simulink model "MicrogridControl"  (R2025b)
settings: Solver=VariableStepAuto  StartTime=0.0  StopTime=8  FixedStep=Ts  RelTol=1e-3
PreLoadFcn:
  | NormalOperation;
  | MicrogridControlParam;
undefined symbols (not defined in the file): base, bessModeInitial, bessSystem, bessVoltage, breakerStatus, DiscIntNeverNeededParam, ee_sli_rtmsupport, event, gcbh, generator, gflInverter, gfmInverter, Inertia, lineInductance, lineResistance, machine, plannedIsland, pmsm, powerLimit, powerQuality, PV, PVInverter, ref, resync, solar, solarInsolationChange, systemFrequency, Ts, windController, windSystem, windTurbine
libraries: nesl_utility x234, ee_lib x174, fl_lib x143, eeGeneralControl x137, simulink x78, eeTransforms x47, slpidlib x23, nesl_utility_internal x12, eePwmGenerator x9, eeSinusoidalMeasurementV2 x9, custom_lib x7, batteryecm_lib x6
(part 12 of 25)

== system MicrogridControl/Wind Farm/Wind Plant Integrated/Detailed/Wind Turbine and Converters ==
  note: Plant
  note: Controller
  pitch : Inport
  Wind_speed : Inport  Port=2
  LVRT : Inport  Port=3
  QRef : Inport  Port=4
  VIBus : Inport  Port=5
  Signal Conditioning : Subsystem
  Wind Controller : Subsystem  mask(Wind Controller){baseVac=Vac, baseImpedance=Vac^2/(plantRating*1000)%base.impedance, basePower=plantRating*1000, inductance=filterInductance, capacitance=0.1, Vdc=baseVoltageDC, frequency=frequency, iMaxPU=iMaxPU, mpptPower=windSystem.mpptPower, mpptWindSpeed=windSystem.mpptWindSpeed, p=p, psim=psim, Rs=Rs, Ld=Ld, Lq=Lq, airDensity=airDensity, turbineRadius=turbineRadius, pitch=pitch, TSR=TSR, cp=cp, wt=wt, rt=wt, Inertia=200, Kp_dc=windController.kpVoltage, Ki_dc=windController.kiVoltage, Kdpi_g=windController.kpId, Kdii_g=windController.kiId, Kqpi_g=windController.kpIq, Kqii_g=windController.kiIq, Kdip_sm=windController.kpMSC, Kdii_sm=windController.kiMSC, Kqip_sm=windController.kpMSC, Kqii_sm=windController.kiMSC}
      mask prompts: baseVac "Base AC Voltage (V)"; baseImpedance "Base Impedance (Ohm)"; basePower "Base Power (W)"; inductance "Filter Inductance (H)"; capacitance "DC bus capacitance (F)"; Vdc "DC bus Voltage (V)"; frequency "System Frequency (Hz)"; iMaxPU "Maximum Current (pu)"; mpptPower "MPPT Power"; mpptWindSpeed "MPPT Wind Speed"; p "Number of pole pairs"; psim "PMSM flux linkage"; Rs "Stator resistance (Ohm)"; Ld "Stator d-axis inductance (H)"; Lq "Stator q-axis inductance (H)"; airDensity "Air Density (kg/m^3)"; turbineRadius "Turbine radius (m)"; pitch "Pitch angle vector (deg)"; cp "Power Coefficient (cp)"; wt "Wind velocity threshold (m/s)"; rt "Rotational velocity threshold (rad/s)"; Inertia "Turbine Inertia (kgm^2)"; Kp_dc "Proportional gain"; Ki_dc "Integral gain"; Kdpi_g "d-axis proportional gain"; Kdii_g "d-axis integrall gain"; Kqpi_g "q-axis proportional gain"; Kqii_g "q-axis integral gain"; Kdip_sm "d-axis proportional gain"; Kdii_sm "d-axis integral gain"; Kqip_sm "q-axis proportional gain"; Kqii_sm "q-axis integral gain"
      mask help: This block implements the control strategy for a Type-4 wind turbine system, which uses a full-scale back-to-back converter to interface the generator with the grid. The controller manages both the machine-side converter (for generator torque and speed control) and the grid-side converter (for active/reactive power regulation and grid compliance). It ensures smooth power transfer, grid code adherence, and dynamic performance under varying wind and grid conditions. The design supports advanced functionalities such as fault ride-through and voltage support.
      mask DialogControl Container9 Prompt: General
      mask DialogControl Container3 Prompt: PMSM Parameters
      mask DialogControl Container4 Prompt: Wind Turbine Parameters
      mask DialogControl Container6 Prompt: Grid Side Converter Controller
      mask DialogControl Container7 Prompt: DC bus voltage controller
      mask DialogControl Container8 Prompt: Current Controller
      mask DialogControl Container10 Prompt: Machine Side Converter Controller
  Wind Plant : Subsystem  mask(Wind Plant){ratedVoltage=Vac, Vdc=baseVoltageDC, capDC=capacitance, airDensity=airDensity, turbineRadius=turbineRadius, pitch=pitch, TSR=TSR, cp=cp, wt=wt, rt=rt, p=p, psim=psim, Rs=Rs, Ld=Ld, Lq=Lq, converterFidelity=Average, fSw=fSw}
      mask prompts: ratedVoltage "Rated voltage on AC side (V)"; Vdc "DC bus violtage (V)"; capDC "DC bus capacitance (F)"; airDensity "Air density (kg/m^3)"; turbineRadius "Turbine radius (m)"; pitch "Pitch angle vector (deg)"; TSR "Tip speed ratio"; cp "Power coefficient table, Cp(beta,TSR)"; wt "Wind velocity threshold (m/s)"; rt "Rotational velocity threshold (rad/s)"; p "Number of pole pairs"; psim "PMSM flux linkage (Wb)"; Rs "Stator resistance (Ohm)"; Ld "Stator d-axis inductance (H)"; Lq "Stator q-axis inductance (H)"; converterFidelity "Converter Fidelity"; fSw "Switching Frequency (kHz)"
      mask help: This block represents the physical interface between the wind turbine and the power converters. It models the electrical and dynamic characteristics of the wind turbine connected to a converter, while expecting an external control signal for operation
      settings: CopyFcn=set_param(gcbh,'LinkStatus','none');
      mask TypeOptions capDC: Back-to-Back Converters/capDC
      mask TypeOptions converterFidelity: Back-to-Back Converters/converterFidelity
      mask Callback converterFidelity: component.mask.setSwitchingFrequency;
      mask TypeOptions fSw: Back-to-Back Converters/fSw
      mask DialogControl Container4 Prompt: General
      mask DialogControl Container5 Prompt: Wind Turbine
      mask DialogControl editWindTurbine Prompt: Edit Wind Turbine Parameters
      mask DialogControl editWindTurbine Callback:
      | blockPath = [gcb,'/','Wind Turbine'];
      | component.mask.openBlock(blockPath);
      mask DialogControl Container6 Prompt: PMSG
      mask DialogControl editMachine Prompt: Edit PMSG Parameters
      mask DialogControl editMachine Callback:
      | blockPath = [gcb,'/','PMSG'];
      | component.mask.openBlock(blockPath);
      mask DialogControl Container7 Prompt: Converter
      mask DialogControl editMSConverter Prompt: Edit machine side converter parameters
      mask DialogControl editMSConverter Callback:
      | converterFidelity = get_param(gcb,'converterFidelity');
      | if strcmp(converterFidelity,'Average')
      |     blockPath = [gcb,'/','Back-to-Back Converters','/',converterFidelity,'/','Machine Side Converter'];
      | else
      |     blockPath = [gcb,'/','Back-to-Back Converters','/',converterFidelity,'/','Machine Side Converter','/','Converter'];
      | end
      | component.mask.openBlock(blockPath);
      mask DialogControl editGSConverter Prompt: Edit grid side converter parameters
      mask DialogControl editGSConverter Callback:
      | converterFidelity = get_param(gcb,'converterFidelity');
      | if strcmp(converterFidelity,'Average')
      |     blockPath = [gcb,'/','Back-to-Back Converters','/',converterFidelity,'/','Grid Side Converter'];
      | else
      |     blockPath = [gcb,'/','Back-to-Back Converters','/',converterFidelity,'/','Grid Side Converter','/','Converter'];
      | end
      | component.mask.openBlock(blockPath);
      mask Display: image('T4wind.png');
  ~ : PMIOPort  Side=Right
  wires:
  Wind Plant/1(PMSM) -> Signal Conditioning/1(PMSM)
  Wind Plant/2(Meas) -> Signal Conditioning/2(Meas)
  Signal Conditioning/5(windSpeed) -> Wind Controller/5(Wind speed)
  Signal Conditioning/4(Vdc) -> Wind Controller/4(vdc)
  Signal Conditioning/3(theta) -> Wind Controller/3(theta)
  Signal Conditioning/2(rotorSpeed) -> Wind Controller/2(w)
  Signal Conditioning/1(iPMSM) -> Wind Controller/1(iPMSM)
  Wind Controller/1(Chopper Control) -> Wind Plant/3(Chopper)
  pitch/1 -> Wind Plant/1(Pitch)
  Wind_speed/1 -> Wind Plant/2(Wind speed)
  Wind Controller/2(SM converter control) -> Wind Plant/4(Machine)
  Wind Controller/3(m_abc) -> Wind Plant/5(Grid)
  LVRT/1 -> Wind Controller/6(LVRT)
  QRef/1 -> Wind Controller/7(QRef)
  VIBus/1 -> Wind Controller/8(VIbus)
  connections:
  Wind Plant/RConn1 -- ~/RConn1

== system MicrogridControl/Wind Farm/Wind Plant Integrated/Simplified/Measurements ==
  Current and Voltage Sensor (Three-Phase)5 : ee_lib/Sensors & Transducers/Current and Voltage Sensor (Three-Phase)  vMeasurementType=ee.enum.vmeasurement.lg  outputUnit=ee.enum.unit.pu  SRated=plantRating*1000 A*V  VRated=Vac V  I_specify=off  I_priority=None  I=[0, 0, 0] A  I_nominal_specify=off  I_nominal_value=1  I_nominal_unit=A  V_specify=off  V_priority=None  V=[0, 0, 0] V  V_nominal_specify=off  V_nominal_value=1  V_nominal_unit=V
      settings: InternalSimscapePortConfiguration="{\"Bottom\":[],\"Left\":[{\"id\":\"N1\",\"label\":\"~1\",\"type\":\"foundation.electrical.three_phase\"}],\"Right\":[{\"id\":\"V_output\",\"label\":\"V\",\"type\":\"output\"},{\"id\":\"I_output\",\"label\":\"I\",\"type\":\"output\"},{\"id\":\"N2\",\"label\":\"~2\",\"type\":\"foundation.electrical.three_phase\"}],\"Top\":[]}"
  Gain : Gain  Gain=1/(plantRating*1000)
  Gain1 : Gain  Gain=1/(plantRating*1000)
  Low-Pass Filter (Discrete or Continuous)1 : eeGeneralControl/Low-Pass Filter (Discrete or Continuous)  K=1  T=0.1  B=inf  A=-inf  init_option=Inherited from block input  x0=0  Ts=-1
  Low-Pass Filter (Discrete or Continuous)2 : eeGeneralControl/Low-Pass Filter (Discrete or Continuous)  K=1  T=0.1  B=inf  A=-inf  init_option=Inherited from block input  x0=0  Ts=-1
  PS-Simulink Converter{,1..3} (4 alike) : nesl_utility/PS-Simulink Converter  PhysicalDomain=network_engine_domain  SubClassName=ps_output  LeftPortType=input  RightPortType=output  PseudoPeriodic=off  Frequencies=[]  VectorFormat=inherit  Unit=inherit  AffineConversion=off
  Power Sensor (Three-Phase) : ee_lib/Sensors & Transducers/Power Sensor (Three-Phase)  load_type=ee.enum.passive.type_balanced.balanced  f0=60 Hz
      settings: InternalSimscapePortConfiguration="{\"Bottom\":[],\"Left\":[{\"id\":\"N1\",\"label\":\"~1\",\"type\":\"foundation.electrical.three_phase\"}],\"Right\":[{\"id\":\"N2\",\"label\":\"~2\",\"type\":\"foundation.electrical.three_phase\"}],\"Top\":[{\"id\":\"Pm\",\"label\":\"P\",\"type\":\"output\"},{\"id\":\"Qm\",\"label\":\"Q\",\"type\":\"output\"}]}"
  In : PMIOPort  Side=Left
  ~ : PMIOPort  Port=2  Side=Right
  P : Outport
  Q : Outport  Port=2
  V : Outport  Port=3
  I : Outport  Port=4
  wires:
  Gain1/1 -> Q/1
  Gain/1 -> P/1
  PS-Simulink Converter3/1 -> I/1
  PS-Simulink Converter2/1 -> V/1
  Low-Pass Filter (Discrete or Continuous)2/1 -> Gain1/1
  Low-Pass Filter (Discrete or Continuous)1/1 -> Gain/1
  PS-Simulink Converter1/1 -> Low-Pass Filter (Discrete or Continuous)2/1
  PS-Simulink Converter/1 -> Low-Pass Filter (Discrete or Continuous)1/1
  connections:
  PS-Simulink Converter3/LConn1 -- Current and Voltage Sensor (Three-Phase)5/RConn2
  Power Sensor (Three-Phase)/RConn1 -- Current and Voltage Sensor (Three-Phase)5/LConn1
  PS-Simulink Converter1/LConn1 -- Power Sensor (Three-Phase)/LConn3
  ~/RConn1 -- Current and Voltage Sensor (Three-Phase)5/RConn3
  In/RConn1 -- Power Sensor (Three-Phase)/LConn1
  PS-Simulink Converter/LConn1 -- Power Sensor (Three-Phase)/LConn2
  PS-Simulink Converter2/LConn1 -- Current and Voltage Sensor (Three-Phase)5/RConn1

== system MicrogridControl/Wind Farm/Wind Plant Integrated1/Detailed/Measurements ==
  Current and Voltage Sensor (Three-Phase)5 : ee_lib/Sensors & Transducers/Current and Voltage Sensor (Three-Phase)  vMeasurementType=ee.enum.vmeasurement.lg  outputUnit=ee.enum.unit.pu  SRated=plantRating*1000 A*V  VRated=Vac V  I_specify=off  I_priority=None  I=[0, 0, 0] A  I_nominal_specify=off  I_nominal_value=1  I_nominal_unit=A  V_specify=off  V_priority=None  V=[0, 0, 0] V  V_nominal_specify=off  V_nominal_value=1  V_nominal_unit=V
      settings: InternalSimscapePortConfiguration="{\"Bottom\":[],\"Left\":[{\"id\":\"N1\",\"label\":\"~1\",\"type\":\"foundation.electrical.three_phase\"}],\"Right\":[{\"id\":\"V_output\",\"label\":\"V\",\"type\":\"output\"},{\"id\":\"I_output\",\"label\":\"I\",\"type\":\"output\"},{\"id\":\"N2\",\"label\":\"~2\",\"type\":\"foundation.electrical.three_phase\"}],\"Top\":[]}"
  Gain : Gain  Gain=1/(plantRating*1000)
  Gain1 : Gain  Gain=1/(plantRating*1000)
  Low-Pass Filter (Discrete or Continuous)1 : eeGeneralControl/Low-Pass Filter (Discrete or Continuous)  K=1  T=0.1  B=inf  A=-inf  init_option=Inherited from block input  x0=0  Ts=-1
  Low-Pass Filter (Discrete or Continuous)2 : eeGeneralControl/Low-Pass Filter (Discrete or Continuous)  K=1  T=0.1  B=inf  A=-inf  init_option=Inherited from block input  x0=0  Ts=-1
  PS-Simulink Converter{,1..3} (4 alike) : nesl_utility/PS-Simulink Converter  PhysicalDomain=network_engine_domain  SubClassName=ps_output  LeftPortType=input  RightPortType=output  PseudoPeriodic=off  Frequencies=[]  VectorFormat=inherit  Unit=inherit  AffineConversion=off
  Power Sensor (Three-Phase) : ee_lib/Sensors & Transducers/Power Sensor (Three-Phase)  load_type=ee.enum.passive.type_balanced.balanced  f0=60 Hz
      settings: InternalSimscapePortConfiguration="{\"Bottom\":[],\"Left\":[{\"id\":\"N1\",\"label\":\"~1\",\"type\":\"foundation.electrical.three_phase\"}],\"Right\":[{\"id\":\"N2\",\"label\":\"~2\",\"type\":\"foundation.electrical.three_phase\"}],\"Top\":[{\"id\":\"Pm\",\"label\":\"P\",\"type\":\"output\"},{\"id\":\"Qm\",\"label\":\"Q\",\"type\":\"output\"}]}"
  In : PMIOPort  Side=Left
  ~ : PMIOPort  Port=2  Side=Right
  P : Outport
  Q : Outport  Port=2
  V : Outport  Port=3
  I : Outport  Port=4
  wires:
  Gain1/1 -> Q/1
  Gain/1 -> P/1
  PS-Simulink Converter3/1 -> I/1
  PS-Simulink Converter2/1 -> V/1
  Low-Pass Filter (Discrete or Continuous)2/1 -> Gain1/1
  Low-Pass Filter (Discrete or Continuous)1/1 -> Gain/1
  PS-Simulink Converter1/1 -> Low-Pass Filter (Discrete or Continuous)2/1
  PS-Simulink Converter/1 -> Low-Pass Filter (Discrete or Continuous)1/1
  connections:
  PS-Simulink Converter3/LConn1 -- Current and Voltage Sensor (Three-Phase)5/RConn2
  Power Sensor (Three-Phase)/RConn1 -- Current and Voltage Sensor (Three-Phase)5/LConn1
  PS-Simulink Converter1/LConn1 -- Power Sensor (Three-Phase)/LConn3
  ~/RConn1 -- Current and Voltage Sensor (Three-Phase)5/RConn3
  In/RConn1 -- Power Sensor (Three-Phase)/LConn1
  PS-Simulink Converter/LConn1 -- Power Sensor (Three-Phase)/LConn2
  PS-Simulink Converter2/LConn1 -- Current and Voltage Sensor (Three-Phase)5/RConn1

== system MicrogridControl/Wind Farm/Wind Plant Integrated1/Detailed/PLL ==
  V : Inport
  I : Inport  Port=2
  PLL & Measurements1 : Subsystem
  VI : Outport
  wires:
  PLL & Measurements1/1(VIbus) -> VI/1
  I/1 -> PLL & Measurements1/2(I)
  V/1 -> PLL & Measurements1/1(V)

== system MicrogridControl/Wind Farm/Wind Plant Integrated1/Detailed/Wind Turbine and Converters ==
  note: Plant
  note: Controller
  pitch : Inport
  Wind_speed : Inport  Port=2
  LVRT : Inport  Port=3
  QRef : Inport  Port=4
  VIBus : Inport  Port=5
  Signal Conditioning : Subsystem
  Wind Controller : Subsystem  mask(Wind Controller){baseVac=Vac, baseImpedance=Vac^2/(plantRating*1000)%base.impedance, basePower=plantRating*1000, inductance=filterInductance, capacitance=0.1, Vdc=baseVoltageDC, frequency=frequency, iMaxPU=iMaxPU, mpptPower=windSystem.mpptPower, mpptWindSpeed=windSystem.mpptWindSpeed, p=p, psim=psim, Rs=Rs, Ld=Ld, Lq=Lq, airDensity=airDensity, turbineRadius=turbineRadius, pitch=pitch, TSR=TSR, cp=cp, wt=wt, rt=wt, Inertia=200, Kp_dc=windController.kpVoltage, Ki_dc=windController.kiVoltage, Kdpi_g=windController.kpId, Kdii_g=windController.kiId, Kqpi_g=windController.kpIq, Kqii_g=windController.kiIq, Kdip_sm=windController.kpMSC, Kdii_sm=windController.kiMSC, Kqip_sm=windController.kpMSC, Kqii_sm=windController.kiMSC}
      mask prompts: baseVac "Base AC Voltage (V)"; baseImpedance "Base Impedance (Ohm)"; basePower "Base Power (W)"; inductance "Filter Inductance (H)"; capacitance "DC bus capacitance (F)"; Vdc "DC bus Voltage (V)"; frequency "System Frequency (Hz)"; iMaxPU "Maximum Current (pu)"; mpptPower "MPPT Power"; mpptWindSpeed "MPPT Wind Speed"; p "Number of pole pairs"; psim "PMSM flux linkage"; Rs "Stator resistance (Ohm)"; Ld "Stator d-axis inductance (H)"; Lq "Stator q-axis inductance (H)"; airDensity "Air Density (kg/m^3)"; turbineRadius "Turbine radius (m)"; pitch "Pitch angle vector (deg)"; cp "Power Coefficient (cp)"; wt "Wind velocity threshold (m/s)"; rt "Rotational velocity threshold (rad/s)"; Inertia "Turbine Inertia (kgm^2)"; Kp_dc "Proportional gain"; Ki_dc "Integral gain"; Kdpi_g "d-axis proportional gain"; Kdii_g "d-axis integrall gain"; Kqpi_g "q-axis proportional gain"; Kqii_g "q-axis integral gain"; Kdip_sm "d-axis proportional gain"; Kdii_sm "d-axis integral gain"; Kqip_sm "q-axis proportional gain"; Kqii_sm "q-axis integral gain"
      mask help: This block implements the control strategy for a Type-4 wind turbine system, which uses a full-scale back-to-back converter to interface the generator with the grid. The controller manages both the machine-side converter (for generator torque and speed control) and the grid-side converter (for active/reactive power regulation and grid compliance). It ensures smooth power transfer, grid code adherence, and dynamic performance under varying wind and grid conditions. The design supports advanced functionalities such as fault ride-through and voltage support.
      mask DialogControl Container9 Prompt: General
      mask DialogControl Container3 Prompt: PMSM Parameters
      mask DialogControl Container4 Prompt: Wind Turbine Parameters
      mask DialogControl Container6 Prompt: Grid Side Converter Controller
      mask DialogControl Container7 Prompt: DC bus voltage controller
      mask DialogControl Container8 Prompt: Current Controller
      mask DialogControl Container10 Prompt: Machine Side Converter Controller
  Wind Plant : Subsystem  mask(Wind Plant){ratedVoltage=Vac, Vdc=baseVoltageDC, capDC=capacitance, airDensity=airDensity, turbineRadius=turbineRadius, pitch=pitch, TSR=TSR, cp=cp, wt=wt, rt=rt, p=p, psim=psim, Rs=Rs, Ld=Ld, Lq=Lq, converterFidelity=Average, fSw=fSw}
      mask prompts: ratedVoltage "Rated voltage on AC side (V)"; Vdc "DC bus violtage (V)"; capDC "DC bus capacitance (F)"; airDensity "Air density (kg/m^3)"; turbineRadius "Turbine radius (m)"; pitch "Pitch angle vector (deg)"; TSR "Tip speed ratio"; cp "Power coefficient table, Cp(beta,TSR)"; wt "Wind velocity threshold (m/s)"; rt "Rotational velocity threshold (rad/s)"; p "Number of pole pairs"; psim "PMSM flux linkage (Wb)"; Rs "Stator resistance (Ohm)"; Ld "Stator d-axis inductance (H)"; Lq "Stator q-axis inductance (H)"; converterFidelity "Converter Fidelity"; fSw "Switching Frequency (kHz)"
      mask help: This block represents the physical interface between the wind turbine and the power converters. It models the electrical and dynamic characteristics of the wind turbine connected to a converter, while expecting an external control signal for operation
      settings: CopyFcn=set_param(gcbh,'LinkStatus','none');
      mask TypeOptions capDC: Back-to-Back Converters/capDC
      mask TypeOptions converterFidelity: Back-to-Back Converters/converterFidelity
      mask Callback converterFidelity: component.mask.setSwitchingFrequency;
      mask TypeOptions fSw: Back-to-Back Converters/fSw
      mask DialogControl Container4 Prompt: General
      mask DialogControl Container5 Prompt: Wind Turbine
      mask DialogControl editWindTurbine Prompt: Edit Wind Turbine Parameters
      mask DialogControl editWindTurbine Callback:
      | blockPath = [gcb,'/','Wind Turbine'];
      | component.mask.openBlock(blockPath);
      mask DialogControl Container6 Prompt: PMSG
      mask DialogControl editMachine Prompt: Edit PMSG Parameters
      mask DialogControl editMachine Callback:
      | blockPath = [gcb,'/','PMSG'];
      | component.mask.openBlock(blockPath);
      mask DialogControl Container7 Prompt: Converter
      mask DialogControl editMSConverter Prompt: Edit machine side converter parameters
      mask DialogControl editMSConverter Callback:
      | converterFidelity = get_param(gcb,'converterFidelity');
      | if strcmp(converterFidelity,'Average')
      |     blockPath = [gcb,'/','Back-to-Back Converters','/',converterFidelity,'/','Machine Side Converter'];
      | else
      |     blockPath = [gcb,'/','Back-to-Back Converters','/',converterFidelity,'/','Machine Side Converter','/','Converter'];
      | end
      | component.mask.openBlock(blockPath);
      mask DialogControl editGSConverter Prompt: Edit grid side converter parameters
      mask DialogControl editGSConverter Callback:
      | converterFidelity = get_param(gcb,'converterFidelity');
      | if strcmp(converterFidelity,'Average')
      |     blockPath = [gcb,'/','Back-to-Back Converters','/',converterFidelity,'/','Grid Side Converter'];
      | else
      |     blockPath = [gcb,'/','Back-to-Back Converters','/',converterFidelity,'/','Grid Side Converter','/','Converter'];
      | end
      | component.mask.openBlock(blockPath);
      mask Display: image('T4wind.png');
  ~ : PMIOPort  Side=Right
  wires:
  Wind Plant/1(PMSM) -> Signal Conditioning/1(PMSM)
  Wind Plant/2(Meas) -> Signal Conditioning/2(Meas)
  Signal Conditioning/5(windSpeed) -> Wind Controller/5(Wind speed)
  Signal Conditioning/4(Vdc) -> Wind Controller/4(vdc)
  Signal Conditioning/3(theta) -> Wind Controller/3(theta)
  Signal Conditioning/2(rotorSpeed) -> Wind Controller/2(w)
  Signal Conditioning/1(iPMSM) -> Wind Controller/1(iPMSM)
  Wind Controller/1(Chopper Control) -> Wind Plant/3(Chopper)
  pitch/1 -> Wind Plant/1(Pitch)
  Wind_speed/1 -> Wind Plant/2(Wind speed)
  Wind Controller/2(SM converter control) -> Wind Plant/4(Machine)
  Wind Controller/3(m_abc) -> Wind Plant/5(Grid)
  LVRT/1 -> Wind Controller/6(LVRT)
  QRef/1 -> Wind Controller/7(QRef)
  VIBus/1 -> Wind Controller/8(VIbus)
  connections:
  Wind Plant/RConn1 -- ~/RConn1

== system MicrogridControl/Wind Farm/Wind Plant Integrated1/Simplified/Measurements ==
  Current and Voltage Sensor (Three-Phase)5 : ee_lib/Sensors & Transducers/Current and Voltage Sensor (Three-Phase)  vMeasurementType=ee.enum.vmeasurement.lg  outputUnit=ee.enum.unit.pu  SRated=plantRating*1000 A*V  VRated=Vac V  I_specify=off  I_priority=None  I=[0, 0, 0] A  I_nominal_specify=off  I_nominal_value=1  I_nominal_unit=A  V_specify=off  V_priority=None  V=[0, 0, 0] V  V_nominal_specify=off  V_nominal_value=1  V_nominal_unit=V
      settings: InternalSimscapePortConfiguration="{\"Bottom\":[],\"Left\":[{\"id\":\"N1\",\"label\":\"~1\",\"type\":\"foundation.electrical.three_phase\"}],\"Right\":[{\"id\":\"V_output\",\"label\":\"V\",\"type\":\"output\"},{\"id\":\"I_output\",\"label\":\"I\",\"type\":\"output\"},{\"id\":\"N2\",\"label\":\"~2\",\"type\":\"foundation.electrical.three_phase\"}],\"Top\":[]}"
  Gain : Gain  Gain=1/(plantRating*1000)
  Gain1 : Gain  Gain=1/(plantRating*1000)
  Low-Pass Filter (Discrete or Continuous)1 : eeGeneralControl/Low-Pass Filter (Discrete or Continuous)  K=1  T=0.1  B=inf  A=-inf  init_option=Inherited from block input  x0=0  Ts=-1
  Low-Pass Filter (Discrete or Continuous)2 : eeGeneralControl/Low-Pass Filter (Discrete or Continuous)  K=1  T=0.1  B=inf  A=-inf  init_option=Inherited from block input  x0=0  Ts=-1
  PS-Simulink Converter{,1..3} (4 alike) : nesl_utility/PS-Simulink Converter  PhysicalDomain=network_engine_domain  SubClassName=ps_output  LeftPortType=input  RightPortType=output  PseudoPeriodic=off  Frequencies=[]  VectorFormat=inherit  Unit=inherit  AffineConversion=off
  Power Sensor (Three-Phase) : ee_lib/Sensors & Transducers/Power Sensor (Three-Phase)  load_type=ee.enum.passive.type_balanced.balanced  f0=60 Hz  config=ee.enum.with_neutral.no  rho=1
      settings: InternalSimscapePortConfiguration="{\"Bottom\":[],\"Left\":[{\"id\":\"N1\",\"label\":\"~1\",\"type\":\"foundation.electrical.three_phase\"}],\"Right\":[{\"id\":\"N2\",\"label\":\"~2\",\"type\":\"foundation.electrical.three_phase\"}],\"Top\":[{\"id\":\"Pm\",\"label\":\"P\",\"type\":\"output\"},{\"id\":\"Qm\",\"label\":\"Q\",\"type\":\"output\"}]}"
  In : PMIOPort  Side=Left
  ~ : PMIOPort  Port=2  Side=Right
  P : Outport
  Q : Outport  Port=2
  V : Outport  Port=3
  I : Outport  Port=4
  wires:
  Gain1/1 -> Q/1
  Gain/1 -> P/1
  PS-Simulink Converter3/1 -> I/1
  PS-Simulink Converter2/1 -> V/1
  Low-Pass Filter (Discrete or Continuous)2/1 -> Gain1/1
  Low-Pass Filter (Discrete or Continuous)1/1 -> Gain/1
  PS-Simulink Converter1/1 -> Low-Pass Filter (Discrete or Continuous)2/1
  PS-Simulink Converter/1 -> Low-Pass Filter (Discrete or Continuous)1/1
  connections:
  PS-Simulink Converter3/LConn1 -- Current and Voltage Sensor (Three-Phase)5/RConn2
  Power Sensor (Three-Phase)/RConn1 -- Current and Voltage Sensor (Three-Phase)5/LConn1
  PS-Simulink Converter1/LConn1 -- Power Sensor (Three-Phase)/LConn3
  ~/RConn1 -- Current and Voltage Sensor (Three-Phase)5/RConn3
  In/RConn1 -- Power Sensor (Three-Phase)/LConn1
  PS-Simulink Converter/LConn1 -- Power Sensor (Three-Phase)/LConn2
  PS-Simulink Converter2/LConn1 -- Current and Voltage Sensor (Three-Phase)5/RConn1

== system MicrogridControl/BESS/BESS Integrated/Detailed/BESS Controller/Grid Following ==
  VRef : Inport
  FRef : Inport  Port=2
  PRef : Inport  Port=3
  QRef : Inport  Port=4
  Mode : Inport  Port=5
  Reset : Inport  Port=6
  In Bus Element3 : Inport  Port=7  PortName=VIBus  Element=Vd
  BusElementIn : Inport  Port=7  PortName=VIBus  Element=Vd
  In Bus Element2 : Inport  Port=7  PortName=VIBus  Element=Vq
  In Bus Element7 : Inport  Port=7  PortName=VIBus  Element=Theta
  BusElementIn1 : Inport  Port=7  PortName=VIBus  Element=Freq
  BusElementIn3 : Inport  Port=7  PortName=VIBus  Element=Id
  BusElementIn4 : Inport  Port=7  PortName=VIBus  Element=Iq
  Constant : Constant  Value=10
  Current_controller : Subsystem
  Inverse Park Transform1 : eeTransforms/Inverse Park Transform  AxisAlignment=Q-axis  PowerInvariant=off
  Reference Current : Subsystem
  Sum2 : Sum  Inputs=|+-
  Terminator : Terminator
  Terminator1 : Terminator
  Unit Delay : UnitDelay  SampleTime=Td  HasFrameUpgradeWarning=on
  Unit Delay1 : UnitDelay  SampleTime=Td  HasFrameUpgradeWarning=on
  Unit Delay2 : UnitDelay  SampleTime=Ts  HasFrameUpgradeWarning=on
  mabc : Outport
  wires:
  QRef/1 -> Reference Current/6(QRef)
  PRef/1 -> Reference Current/5(PRef)
  BusElementIn4/1 -> Current_controller/4(iq)
  BusElementIn3/1 -> Current_controller/2(ipvd)
  BusElementIn1/1 -> Unit Delay1/1
  BusElementIn/1 -> Unit Delay/1
  Unit Delay/1 -> Reference Current/2(V-mag)
  Unit Delay1/1 -> Sum2/2
  Reference Current/1(id_ref) -> Current_controller/1(id-ref)
  Reference Current/2(iq_ref) -> Current_controller/3(iqref)
  Sum2/1 -> Reference Current/3(del f)
  VRef/1 -> Reference Current/1(V_ref)
  FRef/1 -> Sum2/1
  In Bus Element7/1 -> Inverse Park Transform1/2
  In Bus Element3/1 -> Current_controller/5(Vd)
  Current_controller/1(mdq0) -> Inverse Park Transform1/1
  Unit Delay2/1 -> mabc/1
  Inverse Park Transform1/1 -> Unit Delay2/1
  In Bus Element2/1 -> Current_controller/6(Vq)
  Mode/1 -> Terminator/1
  Reset/1 -> Terminator1/1
  Constant/1 -> Reference Current/4(LVRT_iq)

== system MicrogridControl/BESS/BESS Integrated/Detailed/BESS Controller/Grid Forming ==
  VRef : Inport
  FRef : Inport  Port=2
  PRef : Inport  Port=3
  QRef : Inport  Port=4
  Mode : Inport  Port=5
  Reset : Inport  Port=6
  Bus Element In : Inport  Port=7  PortName=VIBus  Element=Vabc
  BusElementIn : Inport  Port=7  PortName=VIBus  Element=Iabc
  Current Limiting : Subsystem
  Grid Voltage Reactive Power Support : Subsystem
  Measurement : Subsystem
      mask Display: image('meas2_1_7_7_2.png');
  Power Control : Subsystem
  Subsystem2 : Subsystem
      settings: PortSchema="{\"entries\":[{\"content\":{\"sides\":[{\"content\":{\"connectorIds\":[\"Out1\"]},\"type\":\"ConnectorPlacement.EquallySpacedRectSide\",\"uuid\":\"7526c1f7-0aba-4355-8bbd-47d168879ecb\"},{\"content\":{\"connectorIds\":[\"In1\",\"In2\"],\"side\":\"RIGHT\"},\"type\":\"ConnectorPlacement.EquallySpacedRectSide\",\"uuid\":\"1dda9693-ec76-4df0-8ad4-aaa83d2574b3\"},{\"content\":{\"side\":\"TOP\"},\"type\":\"ConnectorPlacement.EquallySpacedRectSide\",\"uuid\":\"71ea411b-eb5f-4279-ae23-08ebb3ff1ed6\"}]},\"type\":\"ConnectorPlacement.EquallySpacedConnector\",\"uuid\":\"19864e0c-0998-460d-9705-13c69283d4ec\"}],\"packageUris\":[\"http://schema.mathworks.com/mf0/Connector/R2020b\"],\"version\":\"1.0\"}"
  Terminator : Terminator
  Terminator1 : Terminator
  Terminator2 : Terminator
  VoltageCurrentControl : Subsystem
      settings: PortSchema="{\"entries\":[{\"content\":{\"sides\":[{\"content\":{\"connectorIds\":[\"In1\",\"In2\",\"In3\"]},\"type\":\"ConnectorPlacement.EquallySpacedRectSide\",\"uuid\":\"0bf15a12-7bc0-47e4-89bd-435769673763\"},{\"content\":{\"connectorIds\":[\"Out1\"],\"side\":\"RIGHT\"},\"type\":\"ConnectorPlacement.EquallySpacedRectSide\",\"uuid\":\"44a15d74-8878-4ec6-abe4-be0b1b609519\"},{\"content\":{\"connectorIds\":[\"In4\"],\"side\":\"TOP\"},\"type\":\"ConnectorPlacement.EquallySpacedRectSide\",\"uuid\":\"7a96781e-5638-4b2a-8101-d5785aae9f0f\"}]},\"type\":\"ConnectorPlacement.EquallySpacedConnector\",\"uuid\":\"4b3373ad-cf20-4175-894e-3bd1604dd0ce\"}],\"packageUris\":[\"http://schema.mathworks.com/mf0/Connector/R2020b\"],\"version\":\"1.0\"}"
  mabc : Outport
  wires:
  Reset/1 -> Subsystem2/2(Reset), VoltageCurrentControl/3(Reset)
  Mode/1 -> Power Control/6(CntrlFlag)
  VRef/1 -> Power Control/4(Vref)
  FRef/1 -> Power Control/5(Fref)
  Measurement/4(fmeas) -> Terminator2/1
  Grid Voltage Reactive Power Support/2(Qref) -> Power Control/3(Qref)
  Grid Voltage Reactive Power Support/1(Pref) -> Power Control/2(Pref)
  PRef/1 -> Grid Voltage Reactive Power Support/2(PrefInput)
  QRef/1 -> Grid Voltage Reactive Power Support/3(QrefInput)
  Current Limiting/1(currentLimiting) -> VoltageCurrentControl/1(currentLimiting)
  Power Control/2(activeControl) -> VoltageCurrentControl/2(activeControl)
  Power Control/1(reactiveControl) -> Current Limiting/2(reactiveControl)
  Power Control/3(angle) -> Measurement/3(Angle)
  Measurement/1(measure) -> Grid Voltage Reactive Power Support/1(measure), Power Control/1(measure), VoltageCurrentControl/4(measure), Current Limiting/1(measure)
  Measurement/3(Qmeas) -> Terminator1/1
  Measurement/2(Pmeas) -> Terminator/1
  BusElementIn/1 -> Measurement/2(Igabc)
  Bus Element In/1 -> Measurement/1(Vgabcc)
  VoltageCurrentControl/1(mabc) -> Subsystem2/1(In)
  Subsystem2/1(mabc) -> mabc/1

== system MicrogridControl/BESS/BESS Integrated/Detailed/BESS Plant/Converter ==
  mabc : Inport
  Average : Subsystem  VariantControl=Average
  Switching : Subsystem  VariantControl=Switching
  + : PMIOPort  Side=Left
  - : PMIOPort  Port=2  Side=Left
  ~ : PMIOPort  Port=3  Side=Right

== system MicrogridControl/BESS/BESS Integrated/Detailed/Filter & Measurements/PLL & Measurements ==
  V : Inport
  I : Inport  Port=2
  Measurement1 : Subsystem
  Measurement2 : Subsystem
  Subsystem : Subsystem
  Out Bus Element : Outport  PortName=VIbus  Element=Vq
  Out Bus Element1 : Outport  PortName=VIbus  Element=Vd
  Out Bus Element2 : Outport  PortName=VIbus  Element=Freq
  Out Bus Element3 : Outport  PortName=VIbus  Element=Theta
  Out Bus Element4 : Outport  PortName=VIbus  Element=Vmag
  Out Bus Element5 : Outport  PortName=VIbus  Element=Iq
  Out Bus Element6 : Outport  PortName=VIbus  Element=Id
  Out Bus Element7 : Outport  PortName=VIbus  Element=Iabc
  Out Bus Element8 : Outport  PortName=VIbus  Element=Vabc
  wires:
  Subsystem/6(Id1) -> Out Bus Element6/1
  Subsystem/7(Iq1) -> Out Bus Element5/1
  Measurement1/1(Vg) -> Subsystem/2(Iabc), Out Bus Element7/1
  I/1 -> Measurement1/1(u)
  Subsystem/1(mag) -> Out Bus Element4/1
  Measurement2/1(Vg) -> Subsystem/1(Vabc), Out Bus Element8/1
  Subsystem/4(Vd) -> Out Bus Element1/1
  Subsystem/3(angle) -> Out Bus Element3/1
  Subsystem/5(Vq) -> Out Bus Element/1
  Subsystem/2(freq) -> Out Bus Element2/1
  V/1 -> Measurement2/1(u)

== system MicrogridControl/BESS/BESS Integrated/Simplified/Grid Following/Measurements ==
  Current and Voltage Sensor (Three-Phase)5 : ee_lib/Sensors & Transducers/Current and Voltage Sensor (Three-Phase)  vMeasurementType=ee.enum.vmeasurement.lg  outputUnit=ee.enum.unit.pu  SRated=plantRating*1000 A*V  VRated=Vac V  I_specify=off  I_priority=None  I=[0, 0, 0] A  I_nominal_specify=off  I_nominal_value=1  I_nominal_unit=A  V_specify=off  V_priority=None  V=[0, 0, 0] V  V_nominal_specify=off  V_nominal_value=1  V_nominal_unit=V
      settings: InternalSimscapePortConfiguration="{\"Bottom\":[],\"Left\":[{\"id\":\"N1\",\"label\":\"~1\",\"type\":\"foundation.electrical.three_phase\"}],\"Right\":[{\"id\":\"V_output\",\"label\":\"V\",\"type\":\"output\"},{\"id\":\"I_output\",\"label\":\"I\",\"type\":\"output\"},{\"id\":\"N2\",\"label\":\"~2\",\"type\":\"foundation.electrical.three_phase\"}],\"Top\":[]}"
  Gain1 : Gain  Gain=1/(plantRating*1000)
  Gain2 : Gain  Gain=1/(plantRating*1000)
  Low-Pass Filter (Discrete or Continuous)1 : eeGeneralControl/Low-Pass Filter (Discrete or Continuous)  K=1  T=0.1  B=inf  A=-inf  init_option=Inherited from block input  x0=0  Ts=-1
  Low-Pass Filter (Discrete or Continuous)2 : eeGeneralControl/Low-Pass Filter (Discrete or Continuous)  K=1  T=0.1  B=inf  A=-inf  init_option=Inherited from block input  x0=0  Ts=-1
  PS-Simulink Converter{,1..3} (4 alike) : nesl_utility/PS-Simulink Converter  PhysicalDomain=network_engine_domain  SubClassName=ps_output  LeftPortType=input  RightPortType=output  PseudoPeriodic=off  Frequencies=[]  VectorFormat=inherit  Unit=inherit  AffineConversion=off
  Power Sensor (Three-Phase) : ee_lib/Sensors & Transducers/Power Sensor (Three-Phase)  load_type=ee.enum.passive.type_balanced.balanced  f0=60 Hz
      settings: InternalSimscapePortConfiguration="{\"Bottom\":[],\"Left\":[{\"id\":\"N1\",\"label\":\"~1\",\"type\":\"foundation.electrical.three_phase\"}],\"Right\":[{\"id\":\"N2\",\"label\":\"~2\",\"type\":\"foundation.electrical.three_phase\"}],\"Top\":[{\"id\":\"Pm\",\"label\":\"P\",\"type\":\"output\"},{\"id\":\"Qm\",\"label\":\"Q\",\"type\":\"output\"}]}"
  In : PMIOPort  Side=Left
  ~ : PMIOPort  Port=2  Side=Right
  P : Outport
  Q : Outport  Port=2
  V : Outport  Port=3
  I : Outport  Port=4
  wires:
  Gain2/1 -> Q/1
  Gain1/1 -> P/1
  PS-Simulink Converter3/1 -> I/1
  PS-Simulink Converter2/1 -> V/1
  Low-Pass Filter (Discrete or Continuous)2/1 -> Gain2/1
  Low-Pass Filter (Discrete or Continuous)1/1 -> Gain1/1
  PS-Simulink Converter1/1 -> Low-Pass Filter (Discrete or Continuous)2/1
  PS-Simulink Converter/1 -> Low-Pass Filter (Discrete or Continuous)1/1
  connections:
  PS-Simulink Converter3/LConn1 -- Current and Voltage Sensor (Three-Phase)5/RConn2
  Power Sensor (Three-Phase)/RConn1 -- Current and Voltage Sensor (Three-Phase)5/LConn1
  PS-Simulink Converter1/LConn1 -- Power Sensor (Three-Phase)/LConn3
  ~/RConn1 -- Current and Voltage Sensor (Three-Phase)5/RConn3
  In/RConn1 -- Power Sensor (Three-Phase)/LConn1
  PS-Simulink Converter/LConn1 -- Power Sensor (Three-Phase)/LConn2
  PS-Simulink Converter2/LConn1 -- Current and Voltage Sensor (Three-Phase)5/RConn1

== system MicrogridControl/BESS/BESS Integrated/Simplified/Grid Following/Power Limiter ==
  P : Inport
  SOC : Inport  Port=2
  V : Inport  Port=3
  Add : Sum
  Compare To Constant : simulink/Logic and Bit Operations/Compare To Constant  relop=<=  const=minSOC  OutDataTypeStr=boolean
  Compare To Constant1 : simulink/Logic and Bit Operations/Compare To Constant  relop=>=  const=maxSOC  OutDataTypeStr=boolean
  Constant : Constant  Value=maxSOC
  Constant1 : Constant  Value=0
  Constant2 : Constant  Value=minSOC
  Constant3 : Constant  Value=0
  Constant5 : Constant  Value=minSOC
  Data Type Conversion : DataTypeConversion  OutDataTypeStr=double  SaturateOnIntegerOverflow=off  RndMeth=Floor
  Delay1 : Delay  DelayLength=1
  Divide : Product  Inputs=*/
  Gain : Gain  Gain=-1/(Inf)
  GreaterThan : RelationalOperator  Operator=>  OutDataTypeStr=boolean  RndMeth=Simplest  InputSameDT=off
  GreaterThan1 : RelationalOperator  Operator=<  OutDataTypeStr=boolean  RndMeth=Simplest  InputSameDT=off
  GreaterThan3 : RelationalOperator  Operator=<  OutDataTypeStr=boolean  RndMeth=Simplest  InputSameDT=off
  NOR : Logic  Operator=NOR  IconShape=distinctive  AllPortsSameDT=off  OutDataTypeStr=boolean
  Product : Product
  Scope1 : Scope  NumInputPorts=2
  Scope2 : Scope
  Scope3 : Scope  NumInputPorts=3
  Switch : Switch  Criteria=u2 > Threshold  SaturateOnIntegerOverflow=off  InputSameDT=off
  Switch1 : Switch  Criteria=u2 > Threshold  SaturateOnIntegerOverflow=off  InputSameDT=off
  Switch2 : Switch  Criteria=u2 > Threshold  SaturateOnIntegerOverflow=off  InputSameDT=off
  POut : Outport
  SOCFlag : Outport  Port=2
  wires:
  Product/1 -> POut/1
  Gain/1 -> Add/1
  Data Type Conversion/1 -> Product/2
  NOR/1 -> Data Type Conversion/1
  Compare To Constant1/1 -> NOR/2
  Compare To Constant/1 -> NOR/1
  Add/1 -> Compare To Constant1/1, Compare To Constant/1
  Switch2/1 -> Product/1, Divide/1
  Switch/1 -> Switch2/3, Scope3/3
  SOC/1 -> GreaterThan/1, GreaterThan1/1, Scope2/1, GreaterThan3/1, Add/2
  Divide/1 -> Gain/1
  Delay1/1 -> Divide/2
  V/1 -> Delay1/1
  GreaterThan3/1 -> SOCFlag/1
  Constant5/1 -> GreaterThan3/2
  Constant/1 -> GreaterThan/2
  GreaterThan/1 -> Switch/2
  Constant1/1 -> Switch/1
  Constant2/1 -> GreaterThan1/2
  GreaterThan1/1 -> Switch1/2, Scope1/1
  Constant3/1 -> Switch1/1
  Switch1/1 -> Switch2/1, Scope3/1
  P/1 -> Switch/3, Switch1/3, Switch2/2, Scope3/2

== system MicrogridControl/BESS/BESS Integrated/Simplified/Grid Following/SOC Estimation ==
  I : Inport
  Constant : Constant  Value=0.95
  Gain : Gain  Gain=-1/(100000)
  Integrator (Discrete or Continuous) : eeGeneralControl/Integrator (Discrete or Continuous)  LabelModeActiveChoice=Discrete  IntegratorMethod=Integration: Forward Euler  ExternalReset=level  LimitType=Anti-windup  B=inf  A=-inf  Ts=-1
  SOC : Outport
  wires:
  Integrator (Discrete or Continuous)/1 -> SOC/1
  Gain/1 -> Integrator (Discrete or Continuous)/1
  I/1 -> Gain/1
  Constant/1 -> Integrator (Discrete or Continuous)/3

== system MicrogridControl/BESS/BESS Integrated/Simplified/Grid Forming/Limiter ==
  SOC : Inport
  Compare To Constant : simulink/Logic and Bit Operations/Compare To Constant  relop=<=  const=minSOC  OutDataTypeStr=boolean
  Compare To Constant1 : simulink/Logic and Bit Operations/Compare To Constant  relop=>=  const=maxSOC  OutDataTypeStr=boolean
  Data Type Conversion : DataTypeConversion  OutDataTypeStr=double  SaturateOnIntegerOverflow=off  RndMeth=Floor
  Delay : Delay  DelayLength=1  InputProcessing=Columns as channels (frame based)
  OR : Logic  Operator=OR  AllPortsSameDT=off  OutDataTypeStr=boolean
  Flag : Outport
  wires:
  Delay/1 -> Flag/1
  Data Type Conversion/1 -> Delay/1
  OR/1 -> Data Type Conversion/1
  Compare To Constant1/1 -> OR/2
  Compare To Constant/1 -> OR/1
  SOC/1 -> Compare To Constant1/1, Compare To Constant/1

== system MicrogridControl/BESS/BESS Integrated/Simplified/Grid Forming/Measurements ==
  Current and Voltage Sensor (Three-Phase)5 : ee_lib/Sensors & Transducers/Current and Voltage Sensor (Three-Phase)  vMeasurementType=ee.enum.vmeasurement.lg  outputUnit=ee.enum.unit.pu  SRated=plantRating*1000 A*V  VRated=Vac V  I_specify=off  I_priority=None  I=[0, 0, 0] A  I_nominal_specify=off  I_nominal_value=1  I_nominal_unit=A  V_specify=off  V_priority=None  V=[0, 0, 0] V  V_nominal_specify=off  V_nominal_value=1  V_nominal_unit=V
      settings: InternalSimscapePortConfiguration="{\"Bottom\":[],\"Left\":[{\"id\":\"N1\",\"label\":\"~1\",\"type\":\"foundation.electrical.three_phase\"}],\"Right\":[{\"id\":\"V_output\",\"label\":\"V\",\"type\":\"output\"},{\"id\":\"I_output\",\"label\":\"I\",\"type\":\"output\"},{\"id\":\"N2\",\"label\":\"~2\",\"type\":\"foundation.electrical.three_phase\"}],\"Top\":[]}"
  Gain1 : Gain  Gain=1/(plantRating*1000)
  Gain2 : Gain  Gain=1/(plantRating*1000)
  PS-Simulink Converter{,1..3} (4 alike) : nesl_utility/PS-Simulink Converter  PhysicalDomain=network_engine_domain  SubClassName=ps_output  LeftPortType=input  RightPortType=output  PseudoPeriodic=off  Frequencies=[]  VectorFormat=inherit  Unit=inherit  AffineConversion=off
  Power Sensor (Three-Phase) : ee_lib/Sensors & Transducers/Power Sensor (Three-Phase)  load_type=ee.enum.passive.type_balanced.balanced  f0=60 Hz
      settings: InternalSimscapePortConfiguration="{\"Bottom\":[],\"Left\":[{\"id\":\"N1\",\"label\":\"~1\",\"type\":\"foundation.electrical.three_phase\"}],\"Right\":[{\"id\":\"N2\",\"label\":\"~2\",\"type\":\"foundation.electrical.three_phase\"}],\"Top\":[{\"id\":\"Pm\",\"label\":\"P\",\"type\":\"output\"},{\"id\":\"Qm\",\"label\":\"Q\",\"type\":\"output\"}]}"
  In : PMIOPort  Side=Left
  ~ : PMIOPort  Port=2  Side=Right
  P : Outport
  Q : Outport  Port=2
  V : Outport  Port=3
  I : Outport  Port=4
  wires:
  PS-Simulink Converter1/1 -> Gain2/1
  PS-Simulink Converter/1 -> Gain1/1
  PS-Simulink Converter2/1 -> V/1
  PS-Simulink Converter3/1 -> I/1
  Gain1/1 -> P/1
  Gain2/1 -> Q/1
  connections:
  PS-Simulink Converter2/LConn1 -- Current and Voltage Sensor (Three-Phase)5/RConn1
  PS-Simulink Converter/LConn1 -- Power Sensor (Three-Phase)/LConn2
  In/RConn1 -- Power Sensor (Three-Phase)/LConn1
  ~/RConn1 -- Current and Voltage Sensor (Three-Phase)5/RConn3
  PS-Simulink Converter1/LConn1 -- Power Sensor (Three-Phase)/LConn3
  Power Sensor (Three-Phase)/RConn1 -- Current and Voltage Sensor (Three-Phase)5/LConn1
  PS-Simulink Converter3/LConn1 -- Current and Voltage Sensor (Three-Phase)5/RConn2

== system MicrogridControl/BESS/BESS Integrated/Simplified/Grid Forming/Reference Generator ==
  Mode : Inport
  PRef : Inport  Port=2
  P : Inport  Port=3
  QRef : Inport  Port=4
  Q : Inport  Port=5
  VRef : Inport  Port=6
  V : Inport  Port=7
  Gain : Gain  Gain=efficiency/100
  Gain2 : Gain  Gain=sqrt(3)/Vac
  If : If
  If Action Subsystem : Subsystem  TreatAsAtomicUnit=on
  If Action Subsystem1 : Subsystem  TreatAsAtomicUnit=on
  Merge : Merge
  Merge1 : Merge
  Vt : Outport
  Ph : Outport  Port=2
  wires:
  Gain/1 -> If Action Subsystem/1(PRef)
  Mode/1 -> If/1
  If/1 -> If Action Subsystem/Action
  PRef/1 -> Gain/1, If Action Subsystem1/1(PRef)
  QRef/1 -> If Action Subsystem/3(QRef)
  VRef/1 -> If Action Subsystem1/3(VRef)
  V/1 -> Gain2/1
  If/2 -> If Action Subsystem1/Action
  If Action Subsystem/1(Vt) -> Merge/1
  If Action Subsystem1/1(Vt) -> Merge/2
  If Action Subsystem/2(Ph) -> Merge1/1
  If Action Subsystem1/2(Ph) -> Merge1/2
  Merge1/1 -> Ph/1
  P/1 -> If Action Subsystem/2(P), If Action Subsystem1/2(P)
  Q/1 -> If Action Subsystem/4(Q)
  Gain2/1 -> If Action Subsystem1/4(V)
  Merge/1 -> Vt/1

== system MicrogridControl/BESS/BESS Integrated/Simplified/Grid Forming/SOC Estimation ==
  P : Inport
  Constant : Constant  Value=Vdc
  Constant1 : Constant  Value=initialSOC
  Constant2 : Constant  Value=capacity
  Constant3 : Constant  Value=Inf
  Divide : Product  Inputs=*/
  Divide1 : Product  Inputs=*/
  Gain : Gain  Gain=-plantRating*1000
  Integrator (Discrete or Continuous) : eeGeneralControl/Integrator (Discrete or Continuous)  LabelModeActiveChoice=Discrete  IntegratorMethod=Integration: Forward Euler  ExternalReset=level  LimitType=Anti-windup  B=inf  A=-inf  Ts=-1
  String Compare : StringCompare
  String Constant : StringConstant  String=capacityType
  String Constant1 : StringConstant  String="\"Fixed\""
  Switch : Switch  Criteria=u2 > Threshold  SaturateOnIntegerOverflow=off  InputSameDT=off
  Meas : Outport
  wires:
  Gain/1 -> Divide/1
  P/1 -> Gain/1
  Constant/1 -> Divide/2
  Divide/1 -> Divide1/1
  Constant1/1 -> Integrator (Discrete or Continuous)/3
  Integrator (Discrete or Continuous)/1 -> Meas/1
  String Constant/1 -> String Compare/1
  String Constant1/1 -> String Compare/2
  String Compare/1 -> Switch/2
  Switch/1 -> Divide1/2
  Divide1/1 -> Integrator (Discrete or Continuous)/1
  Constant2/1 -> Switch/1
  Constant3/1 -> Switch/3

== system MicrogridControl/BESS/BESS Integrated1/Detailed/BESS Controller/Grid Following ==
  VRef : Inport
  FRef : Inport  Port=2
  PRef : Inport  Port=3
  QRef : Inport  Port=4
  Mode : Inport  Port=5
  Reset : Inport  Port=6
  In Bus Element3 : Inport  Port=7  PortName=VIBus  Element=Vd
  BusElementIn : Inport  Port=7  PortName=VIBus  Element=Vd
  In Bus Element2 : Inport  Port=7  PortName=VIBus  Element=Vq
  In Bus Element7 : Inport  Port=7  PortName=VIBus  Element=Theta
  BusElementIn1 : Inport  Port=7  PortName=VIBus  Element=Freq
  BusElementIn3 : Inport  Port=7  PortName=VIBus  Element=Id
  BusElementIn4 : Inport  Port=7  PortName=VIBus  Element=Iq
  Constant : Constant  Value=10
  Current_controller : Subsystem
  Inverse Park Transform1 : eeTransforms/Inverse Park Transform  AxisAlignment=Q-axis  PowerInvariant=off
  Reference Current : Subsystem
  Sum2 : Sum  Inputs=|+-
  Terminator : Terminator
  Terminator1 : Terminator
  Unit Delay : UnitDelay  SampleTime=Td  HasFrameUpgradeWarning=on
  Unit Delay1 : UnitDelay  SampleTime=Td  HasFrameUpgradeWarning=on
  Unit Delay2 : UnitDelay  SampleTime=Ts  HasFrameUpgradeWarning=on
  mabc : Outport
  wires:
  QRef/1 -> Reference Current/6(QRef)
  PRef/1 -> Reference Current/5(PRef)
  BusElementIn4/1 -> Current_controller/4(iq)
  BusElementIn3/1 -> Current_controller/2(ipvd)
  BusElementIn1/1 -> Unit Delay1/1
  BusElementIn/1 -> Unit Delay/1
  Unit Delay/1 -> Reference Current/2(V-mag)
  Unit Delay1/1 -> Sum2/2
  Reference Current/1(id_ref) -> Current_controller/1(id-ref)
  Reference Current/2(iq_ref) -> Current_controller/3(iqref)
  Sum2/1 -> Reference Current/3(del f)
  VRef/1 -> Reference Current/1(V_ref)
  FRef/1 -> Sum2/1
  In Bus Element7/1 -> Inverse Park Transform1/2
  In Bus Element3/1 -> Current_controller/5(Vd)
  Current_controller/1(mdq0) -> Inverse Park Transform1/1
  Unit Delay2/1 -> mabc/1
  Inverse Park Transform1/1 -> Unit Delay2/1
  In Bus Element2/1 -> Current_controller/6(Vq)
  Mode/1 -> Terminator/1
  Reset/1 -> Terminator1/1
  Constant/1 -> Reference Current/4(LVRT_iq)

== system MicrogridControl/BESS/BESS Integrated1/Detailed/BESS Controller/Grid Forming ==
  VRef : Inport
  FRef : Inport  Port=2
  PRef : Inport  Port=3
  QRef : Inport  Port=4
  Mode : Inport  Port=5
  Reset : Inport  Port=6
  Bus Element In : Inport  Port=7  PortName=VIBus  Element=Vabc
  BusElementIn : Inport  Port=7  PortName=VIBus  Element=Iabc
  Current Limiting : Subsystem
  Grid Voltage Reactive Power Support : Subsystem
  Measurement : Subsystem
      mask Display: image('meas2_1_7_7_2_1.png');
  Power Control : Subsystem
  Subsystem2 : Subsystem
      settings: PortSchema="{\"entries\":[{\"content\":{\"sides\":[{\"content\":{\"connectorIds\":[\"Out1\"]},\"type\":\"ConnectorPlacement.EquallySpacedRectSide\",\"uuid\":\"7526c1f7-0aba-4355-8bbd-47d168879ecb\"},{\"content\":{\"connectorIds\":[\"In1\",\"In2\"],\"side\":\"RIGHT\"},\"type\":\"ConnectorPlacement.EquallySpacedRectSide\",\"uuid\":\"1dda9693-ec76-4df0-8ad4-aaa83d2574b3\"},{\"content\":{\"side\":\"TOP\"},\"type\":\"ConnectorPlacement.EquallySpacedRectSide\",\"uuid\":\"71ea411b-eb5f-4279-ae23-08ebb3ff1ed6\"}]},\"type\":\"ConnectorPlacement.EquallySpacedConnector\",\"uuid\":\"19864e0c-0998-460d-9705-13c69283d4ec\"}],\"packageUris\":[\"http://schema.mathworks.com/mf0/Connector/R2020b\"],\"version\":\"1.0\"}"
  Terminator : Terminator
  Terminator1 : Terminator
  Terminator2 : Terminator
  VoltageCurrentControl : Subsystem
      settings: PortSchema="{\"entries\":[{\"content\":{\"sides\":[{\"content\":{\"connectorIds\":[\"In1\",\"In2\",\"In3\"]},\"type\":\"ConnectorPlacement.EquallySpacedRectSide\",\"uuid\":\"0bf15a12-7bc0-47e4-89bd-435769673763\"},{\"content\":{\"connectorIds\":[\"Out1\"],\"side\":\"RIGHT\"},\"type\":\"ConnectorPlacement.EquallySpacedRectSide\",\"uuid\":\"44a15d74-8878-4ec6-abe4-be0b1b609519\"},{\"content\":{\"connectorIds\":[\"In4\"],\"side\":\"TOP\"},\"type\":\"ConnectorPlacement.EquallySpacedRectSide\",\"uuid\":\"7a96781e-5638-4b2a-8101-d5785aae9f0f\"}]},\"type\":\"ConnectorPlacement.EquallySpacedConnector\",\"uuid\":\"4b3373ad-cf20-4175-894e-3bd1604dd0ce\"}],\"packageUris\":[\"http://schema.mathworks.com/mf0/Connector/R2020b\"],\"version\":\"1.0\"}"
  mabc : Outport
  wires:
  Reset/1 -> Subsystem2/2(Reset), VoltageCurrentControl/3(Reset)
  Mode/1 -> Power Control/6(CntrlFlag)
  VRef/1 -> Power Control/4(Vref)
  FRef/1 -> Power Control/5(Fref)
  Measurement/4(fmeas) -> Terminator2/1
  Grid Voltage Reactive Power Support/2(Qref) -> Power Control/3(Qref)
  Grid Voltage Reactive Power Support/1(Pref) -> Power Control/2(Pref)
  PRef/1 -> Grid Voltage Reactive Power Support/2(PrefInput)
  QRef/1 -> Grid Voltage Reactive Power Support/3(QrefInput)
  Current Limiting/1(currentLimiting) -> VoltageCurrentControl/1(currentLimiting)
  Power Control/2(activeControl) -> VoltageCurrentControl/2(activeControl)
  Power Control/1(reactiveControl) -> Current Limiting/2(reactiveControl)
  Power Control/3(angle) -> Measurement/3(Angle)
  Measurement/1(measure) -> Grid Voltage Reactive Power Support/1(measure), Power Control/1(measure), VoltageCurrentControl/4(measure), Current Limiting/1(measure)
  Measurement/3(Qmeas) -> Terminator1/1
  Measurement/2(Pmeas) -> Terminator/1
  BusElementIn/1 -> Measurement/2(Igabc)
  Bus Element In/1 -> Measurement/1(Vgabcc)
  VoltageCurrentControl/1(mabc) -> Subsystem2/1(In)
  Subsystem2/1(mabc) -> mabc/1
